simulink model "test_vibration_equivalence_harness"  (R2026a)
settings: Solver=FixedStepAuto  StopTime=StopTime_harness  FixedStep=Ts_harness
values from neighbouring files (symbols this model uses):
  Ts_harness = 0.004    [check_item5_simulink_vs_replay_equivalence.m]
settings Model: Creator=Edison Altamirano  LastModifiedBy=Edison Altamirano

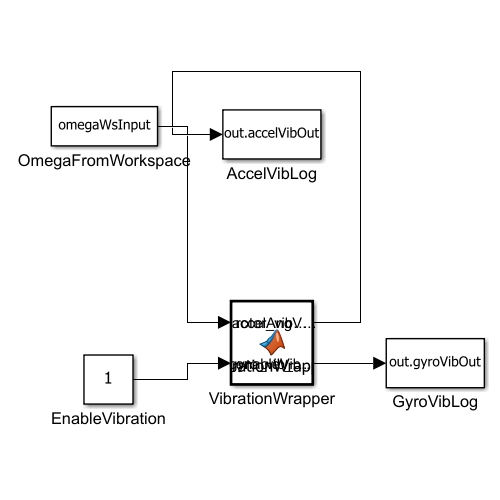
[thumbnail: Simulink's stored preview of the top-level diagram]
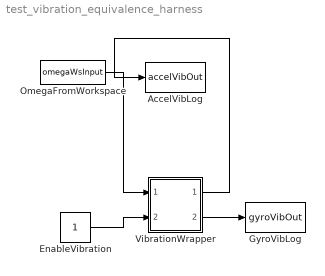
== system test_vibration_equivalence_harness ==
  AccelVibLog : ToWorkspace  VariableName=accelVibOut  SampleTime=Ts_harness
  EnableVibration : Constant
  GyroVibLog : ToWorkspace  VariableName=gyroVibOut  SampleTime=Ts_harness
  OmegaFromWorkspace : FromWorkspace  VariableName=omegaWsInput  SampleTime=Ts_harness  Interpolate=off  ZeroCross=off  OutputAfterFinalValue=Holding final value
  VibrationWrapper : MATLAB Function  TreatAsAtomicUnit=on
  wires:
  OmegaFromWorkspace/1 -> VibrationWrapper/1(rotorAngVel_radps)
  EnableVibration/1 -> VibrationWrapper/2(enableVibration)
  VibrationWrapper/1(accel_vib_mps2) -> AccelVibLog/1
  VibrationWrapper/2(gyro_vib_radps) -> GyroVibLog/1

== matlab function test_vibration_equivalence_harness/VibrationWrapper ==
  data: rotorAngVel_radps input; accel_vib_mps2 output; enableVibration input; gyro_vib_radps output
function [accel_vib_mps2, gyro_vib_radps] = VibrationWrapper(rotorAngVel_radps, enableVibration)
%#codegen
[accel_vib_mps2, gyro_vib_radps] = ANELLO_X3_Vibration_LevelA_fcn(rotorAngVel_radps, enableVibration);
end
